simulink model "sltestProjectorFanSpeedExample"  (R2017a)
settings: Solver=ode15s  StartTime=0.0  StopTime=200  RelTol=1e-3  EnableMultiTasking=on
PreLoadFcn:
  | Simscape_Thermal_Projector_Parameters;
undefined symbols (not defined in the file or in its folder): Fan_Flow, Initial_Temp, Lamp_Power
libraries: fl_lib x13, nesl_utility x4
settings Model: Creator=The MathWorks, Inc.  LastModifiedBy=The MathWorks, Inc.
settings DataIOCC: LimitDataPoints=on  SaveFormat=Array
settings OptimizationCC: ExpressionDepthLimit=2147483647  InitFltsAndDblsToZero=on  LifeSpan=inf
settings DebuggingCC: AlgebraicLoopMsg=none  SaveWithParameterizedLinksMsg=none  UnderspecifiedInitializationDetection=Classic  MergeDetectMultiDrivingBlocksExec=none  SignalResolutionControl=TryResolveAllWithWarning  MultiTaskDSMMsg=warning  MultiTaskCondExecSysMsg=none  FcnCallInpInsideContextMsg=warning  AllowSymbolicDim=off  StateNameClashWarn=warning  SFUnexpectedBacktrackingDiag=warning  SFNoUnconditionalDefaultTransitionDiag=warning  SFExecutionAtInitializationDiag=none
settings HardwareCC: ProdBitPerPointer=32  ProdBitPerSizeT=32  ProdBitPerPtrDiffT=32  ProdLargestAtomicFloat=None  ProdIntDivRoundTo=Undefined  ProdEndianess=Unspecified  ProdWordSize=32  ProdHWDeviceType=32-bit Generic  TargetBitPerLong=64  TargetBitPerPointer=64  TargetBitPerSizeT=64  TargetBitPerPtrDiffT=64  TargetLongLongMode=on  TargetIntDivRoundTo=Zero  TargetEndianess=LittleEndian  TargetWordSize=64  TargetHWDeviceType=MATLAB Host  ProdEqTarget=off
settings ModelReferenceCC: PropagateSignalLabelsOutOfModel=off
settings SFSimCC: SimParseCustomCode=off
settings RTWCC: SystemTargetFile=rsim.tlc  TemplateMakefile=rsim_default_tmf  Description=Rapid Simulation Target
settings ConfigComp: CovMetricSettings=dw  CovHtmlReporting=on  CovSaveCumulativeToWorkspaceVar=on  CovSaveSingleToWorkspaceVar=on  CovExternalEMLEnable=off

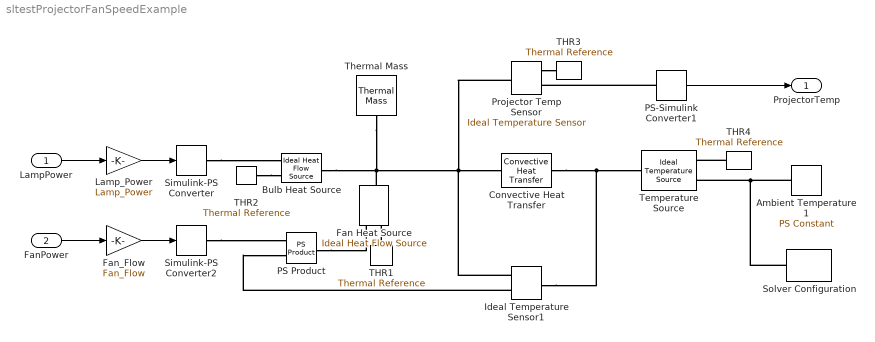
== system sltestProjectorFanSpeedExample ==
  LampPower : Inport
  FanPower : Inport  Port=2
  Ambient Temperature1 : fl_lib/Physical Signals/Sources/PS Constant  constant=Ambient_Temp
  Bulb Heat Source : fl_lib/Thermal/Thermal Sources/Ideal Heat Flow Source
      settings: SourceProductName=Simscape  SourceProductBaseCode=SS
  Convective Heat Transfer : fl_lib/Thermal/Thermal Elements/Convective Heat Transfer  area=Surface_Area m^2  heat_tr_coeff=k_convection W/m^2/K  Q_specify=off  Q_priority=High  Q=0 J/s  Q_nominal_specify=off  Q_nominal_unit=J/s  Q_nominal_value=1  T_specify=off  T_priority=High  T=0 K  T_nominal_specify=off  T_nominal_unit=K  T_nominal_value=1
  Fan Heat Source : fl_lib/Thermal/Thermal Sources/Ideal Heat Flow Source
      settings: SourceProductName=Simscape  SourceProductBaseCode=SS
  Fan_Flow : Gain  Gain=Fan_Flow
  Ideal Temperature Sensor1 : fl_lib/Thermal/Thermal Sensors/Ideal Temperature Sensor
      settings: SourceProductName=Simscape  SourceProductBaseCode=SS
  Lamp_Power : Gain  Gain=Lamp_Power
  PS Product : fl_lib/Physical Signals/Functions/PS Product
      settings: SourceProductName=Simscape
  PS-Simulink Converter1 : nesl_utility/PS-Simulink Converter  PhysicalDomain=network_engine_domain  SubClassName=ps_output  LeftPortType=input  RightPortType=output  PseudoPeriodic=off  Frequencies=[]  Unit=degC  AffineConversion=on
  Projector Temp Sensor : fl_lib/Thermal/Thermal Sensors/Ideal Temperature Sensor
      settings: SourceProductName=Simscape  SourceProductBaseCode=SS
  Simulink-PS Converter : nesl_utility/Simulink-PS Converter  PhysicalDomain=network_engine_domain  SubClassName=ps_input  LeftPortType=input  RightPortType=output  PseudoPeriodic=off  Frequencies=[]  NoiseDistribution=none  NoiseParameters=[]  Unit=J/s  AffineConversion=off  FilteringAndDerivatives=zero  SimscapeFilterOrder=1  InputFilterTimeConstant=.001  UdotUserProvided=0
  Simulink-PS Converter2 : nesl_utility/Simulink-PS Converter  PhysicalDomain=network_engine_domain  SubClassName=ps_input  LeftPortType=input  RightPortType=output  PseudoPeriodic=off  Frequencies=[]  NoiseDistribution=none  NoiseParameters=[]  Unit=W/K  AffineConversion=off  FilteringAndDerivatives=zero  SimscapeFilterOrder=1  InputFilterTimeConstant=.001  UdotUserProvided=0
  Solver Configuration : nesl_utility/Solver Configuration  PhysicalDomain=network_engine_domain  SubClassName=solver  LeftPortType=input  RightPortType=generic  Accelerate=off  Tones=[]  Harmonics=[]  SimulateNoise=off  Profile=off  UseLocalSampling=off  EnableSwitchedLinearOptims=on  FrequencyDomain=off  UseCCode=off  RelTol=0.001  AbsTol=1e-06  MinStep=1e-09  ToWorkspace=off  RevertToSquareIcSolve=off  NumHomotopyIterations=100  PhasorMode=off  PhasorModeNumHarmonics=1  OverrideAbsTol=off  DoDC=off  ResidualTolerance=1e-9  UseLocalSolver=off  LocalSolverChoice=NE_BACKWARD_EULER_ADVANCER  LocalSolverSampleTime=.001  DoFixedCost=off  MaxNonlinIter=12  MaxModeIter=2  LinearAlgebra=Sparse  DelaysMemoryBudget=1024  AutomaticFiltering=on  FilteringTimeConstant=0.001
  THR{1..4} (4 alike) : fl_lib/Thermal/Thermal Elements/Thermal Reference
  Temperature Source : fl_lib/Thermal/Thermal Sources/Ideal Temperature Source
      settings: SourceProductName=Simscape  SourceProductBaseCode=SS
  Thermal Mass : fl_lib/Thermal/Thermal Elements/Thermal Mass  mass=m kg  sp_heat=Cp J/kg/K  T_specify=on  T_priority=High  T=Initial_Temp K  T_nominal_specify=off  T_nominal_unit=K  T_nominal_value=1  Q_specify=off  Q_priority=High  Q=0 J/s  Q_nominal_specify=off  Q_nominal_unit=J/s  Q_nominal_value=1
  ProjectorTemp : Outport
  wires:
  PS-Simulink Converter1/1 -> ProjectorTemp/1
  Fan_Flow/1 -> Simulink-PS Converter2/1
  Lamp_Power/1 -> Simulink-PS Converter/1
  LampPower/1 -> Lamp_Power/1
  FanPower/1 -> Fan_Flow/1
  connections:
  Bulb Heat Source/LConn1 -- Ideal Temperature Sensor1/RConn1 -- Projector Temp Sensor/LConn1 -- Convective Heat Transfer/LConn1 -- Fan Heat Source/LConn1 -- Thermal Mass/LConn1
  Convective Heat Transfer/RConn1 -- Ideal Temperature Sensor1/LConn1 -- Temperature Source/LConn1
  Projector Temp Sensor/RConn1 -- THR3/LConn1
  PS-Simulink Converter1/LConn1 -- Projector Temp Sensor/RConn2
  Simulink-PS Converter/RConn1 -- Bulb Heat Source/RConn1
  Simulink-PS Converter2/RConn1 -- PS Product/LConn2
  PS Product/RConn1 -- Fan Heat Source/RConn1
  THR1/LConn1 -- Fan Heat Source/RConn2
  THR2/LConn1 -- Bulb Heat Source/RConn2
  Ideal Temperature Sensor1/RConn2 -- PS Product/LConn1
  THR4/LConn1 -- Temperature Source/RConn2
  Ambient Temperature1/RConn1 -- Solver Configuration/RConn1 -- Temperature Source/RConn1
